simulink model "model"  (R2024b)
settings: Solver=VariableStepAuto  StartTime=0.0  StopTime=100  FixedStep=0.01  RelTol=1e-3
settings Model: Creator=student  LastModifiedBy=SzymonWysoglad
settings DataIOCC: ExternalInput=x_sim, y_sim
settings RTWCC: GPUComputeCapability=3.5

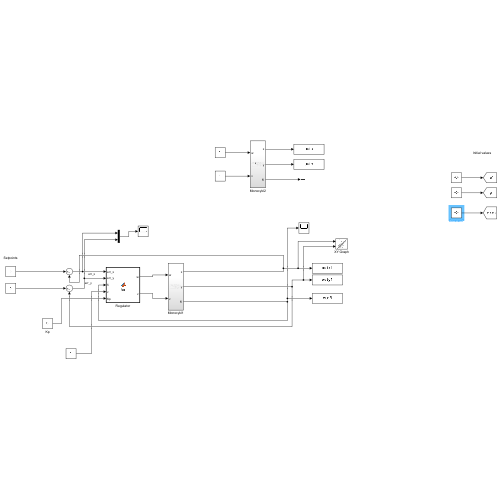
[thumbnail: Simulink's stored preview of the top-level diagram]
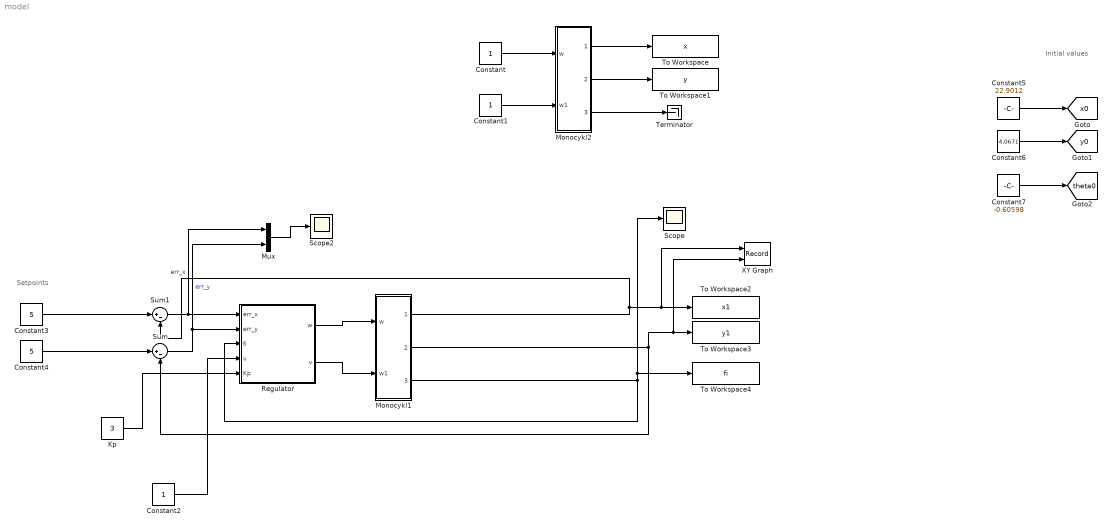
== system model ==
  note: Initial values
  note: Setpoints
  Constant : Constant
  Constant1 : Constant
  Constant2 : Constant
  Constant3 : Constant  Value=5
  Constant4 : Constant  Value=5
  Constant5 : Constant  Value=22.9012
  Constant6 : Constant  Value=4.0671
  Constant7 : Constant  Value=-0.60598
  Kp : Constant  Value=3
  Monocykl1 : Subsystem
  Monocykl2 : Subsystem
  Mux : Mux  Inputs=2
  Regulator : MATLAB Function  TreatAsAtomicUnit=on
  Scope : Scope
  Scope2 : Scope
  Sum : Sum  Inputs=|+-
  Sum1 : Sum  Inputs=|+-
  Terminator : Terminator
  To Workspace : ToWorkspace  VariableName=x  SampleTime=-1
  To Workspace1 : ToWorkspace  VariableName=y  SampleTime=-1
  To Workspace2 : ToWorkspace  VariableName=x1  SampleTime=-1
  To Workspace3 : ToWorkspace  VariableName=y1  SampleTime=-1
  To Workspace4 : ToWorkspace  VariableName=fi  SampleTime=-1
  XY Graph : Record  FileSettingsInternal="{\"entries\":[{\"content\":{\"excelSettings\":{\"content\":{},\"type\":\"Streamout.ExcelSettings\"}},\"type\":\"Streamout.FileSettingStorage\",\"uuid\":\"\"}],\"packageUris\":[\"http:\\/\\/schema.mathworks.com\\/mf0\\/streamout_blocks\\/R2020a\"],\"version\":\"1.0\"}"  Layout=[1 1]  SignalsInternal="{\"entries\":[{\"content\":{\"signals\":[{\"content\":{\"blockPath\":[],\"dimensions\":[1],\"domain\":\"\",\"lineColor\":\"#a2142f\",\"plots\":[ 1 ],\"port\":1,\"sid\":[\"\"],\"signalID\":1,\"signalName\":\"Monocykl1:1\"},\"type\":\"RecordBlkView.Signal\",\"uuid\":\"\"},{\"content\":{\"blockPath\":[],\"dimensions\":[1],\"domain\":\"\",\"lineColor\":\"#139fff\",\"plots\":[ 1 ],\"port\":2,\"sid\":[\"\"],\"signalID\":2,\"signalName\":\"Monocykl1:2\"},\"type\":\"RecordBlkView.Signal\",\"uuid\":\"\"}]},\"type\":\"RecordBlkView.InputSignals\",\"uuid\":\"\"}],\"packageUris\":[\"http:\\/\\/schema.mathworks.com\\/mf0\\/streamout_blocks\\/R2020a\"],\"version\":\"1.0\"}"  VisualizationBindings="{\"xyplotplugin\":{\"info\":[{\"series\":[{\"bindingParametersList\":[{\"parameter\":\"X-Axis\",\"signalID\":1,\"signalName\":\"Monocykl1:1\"},{\"parameter\":\"Y-Axis\",\"signalID\":2,\"signalName\":\"Monocykl1:2\"}],\"seriesID\":0}],\"subplotID\":1}]}}"  CompatibilityTag=XY
  tag scope: theta0=global, x0=global, y0=global
  wires:
  Monocykl2/1(Out1) -> To Workspace/1
  Monocykl2/2(Out2) -> To Workspace1/1
  Constant/1 -> Monocykl2/1(w)
  Constant1/1 -> Monocykl2/2(w1)
  Monocykl1/2(Out2) -> XY Graph/2, To Workspace3/1, Sum/2
  Monocykl1/1(Out1) -> Sum1/2, To Workspace2/1, XY Graph/1
  Sum1/1 -> Mux/1, Regulator/1(err_x)  "err_x"
  Constant3/1 -> Sum1/1
  Regulator/1(w) -> Monocykl1/1(w)
  Sum/1 -> Mux/2, Regulator/2(err_y)  "err_y"
  Constant2/1 -> Regulator/4("v ")
  Monocykl1/3(theta) -> Scope/1, To Workspace4/1, Regulator/3(fi)
  Regulator/2(v) -> Monocykl1/2(w1)
  Mux/1 -> Scope2/1
  Constant4/1 -> Sum/1
  Kp/1 -> Regulator/5(Kp)
  Constant6/1 -> [y0]
  Constant5/1 -> [x0]
  Constant7/1 -> [theta0]
  Monocykl2/3(theta) -> Terminator/1

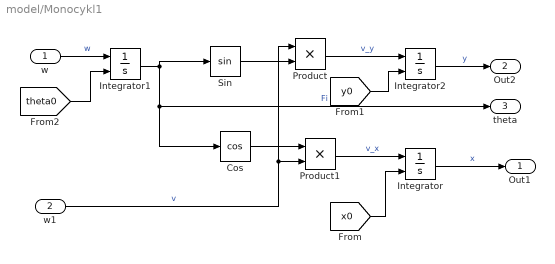
== system model/Monocykl1 ==
  w : Inport
  w1 : Inport  Port=2
  Cos : Trigonometry  Operator=cos
  Integrator : Integrator  InitialConditionSource=external
  Integrator1 : Integrator  InitialConditionSource=external
  Integrator2 : Integrator  InitialConditionSource=external
  Product : Product
  Product1 : Product
  Sin : Trigonometry
  Out1 : Outport
  Out2 : Outport  Port=2
  theta : Outport  Port=3
  wires:
  w1/1 -> Product1/2, Product/1  "v"
  w/1 -> Integrator1/1  "w"
  Integrator1/1 -> Sin/1, Cos/1, theta/1  "Fi"
  Cos/1 -> Product1/1
  Sin/1 -> Product/2
  Product1/1 -> Integrator/1  "v_x"
  Product/1 -> Integrator2/1  "v_y"
  Integrator/1 -> Out1/1  "x"
  Integrator2/1 -> Out2/1  "y"
  [x0] -> Integrator/2
  [y0] -> Integrator2/2
  [theta0] -> Integrator1/2

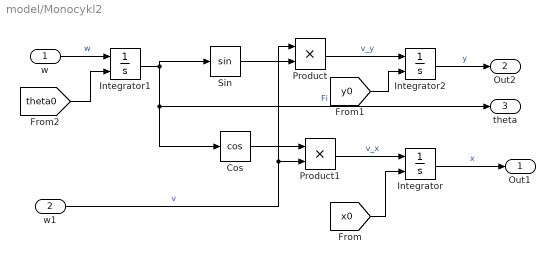
== system model/Monocykl2 ==
  w : Inport
  w1 : Inport  Port=2
  Cos : Trigonometry  Operator=cos
  Integrator : Integrator  InitialConditionSource=external
  Integrator1 : Integrator  InitialConditionSource=external
  Integrator2 : Integrator  InitialConditionSource=external
  Product : Product
  Product1 : Product
  Sin : Trigonometry
  Out1 : Outport
  Out2 : Outport  Port=2
  theta : Outport  Port=3
  wires:
  w1/1 -> Product1/2, Product/1  "v"
  w/1 -> Integrator1/1  "w"
  Integrator1/1 -> Sin/1, Cos/1, theta/1  "Fi"
  Cos/1 -> Product1/1
  Sin/1 -> Product/2
  Product1/1 -> Integrator/1  "v_x"
  Product/1 -> Integrator2/1  "v_y"
  Integrator/1 -> Out1/1  "x"
  Integrator2/1 -> Out2/1  "y"
  [x0] -> Integrator/2
  [y0] -> Integrator2/2
  [theta0] -> Integrator1/2

== matlab function model/Regulator ==
  data: err_x input; w output; err_y input; fi input; v output; v input; Kp input
function [w, v] = fcn(err_x, err_y, fi, v, Kp)
    eps = 0.1;
    desir_fi = atan2(err_y, err_x);

    % Jeśli błąd jest bardzo mały, zatrzymaj ruch
    if (abs(err_y) < eps && abs(err_x) < eps)
        w = 0;
        v = 0;
        return;
    end


    fi_diff = mod(fi - desir_fi, 2*pi);
    if (fi_diff > pi)
        w = Kp;  % obrot w lewo
    else
        w = -Kp; % obrot w prawo
    end
    
end
